simulink model "LP6"  (R2021a)
settings: Solver=VariableStepAuto  StartTime=0.0  StopTime=10.0  RelTol=1e-3
settings Model: Creator=Rubina  LastModifiedBy=Rubina

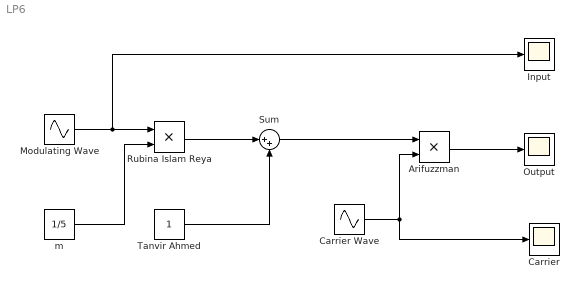
== system LP6 ==
  Arifuzzman : Product
  Carrier : Scope
  Carrier Wave : Sin  SampleTime=0
  Input : Scope
  Modulating Wave : Sin  Amplitude=5  Frequency=2*pi*25  SampleTime=1/5000
  Output : Scope
  Rubina Islam Reya : Product
  Sum : Sum  Inputs=|++
  Tanvir Ahmed : Constant
  m : Constant  Value=1/5
  wires:
  Modulating Wave/1 -> Input/1, Rubina Islam Reya/1
  m/1 -> Rubina Islam Reya/2
  Rubina Islam Reya/1 -> Sum/1
  Tanvir Ahmed/1 -> Sum/2
  Sum/1 -> Arifuzzman/1
  Carrier Wave/1 -> Carrier/1, Arifuzzman/2
  Arifuzzman/1 -> Output/1
